simulink model "rtp_vector"  (R2024a)
settings: Solver=VariableStepAuto  StartTime=0.0  StopTime=4096*2  RelTol=1e-3
PostLoadFcn:
  | load filters
values from neighbouring files (symbols this model uses):
  narrow_filter = [180 89 -80 -391 -720 -834 -478 505 2063 3896 5535 6504]    [filters.mat]
  wide_filter = [-21 -249 319 -78 -511 977 -610 -844 2574 -2754 -1066 18539]    [filters.mat]
undefined symbols (not defined in the file or in its folder): None, S, vsva2197, xcvc1902
libraries: aieDSP x1, simulink x1, vmcUtilities x1, aieUtilities x1, dspobslib x1
settings Model: PauseTimes=511  Creator=abehbood  LastModifiedBy=robg
settings SolverCC: AlgebraicLoopSolver=TrustRegion
settings DebuggingCC: UnconnectedInputMsg=warning  UnconnectedOutputMsg=warning  UnconnectedLineMsg=warning
settings ModelReferenceCC: EnableRefExpFcnMdlSchedulingChecks=on
settings RTWCC: GPUComputeCapability=3.5  DLArmComputeVersion=19.05

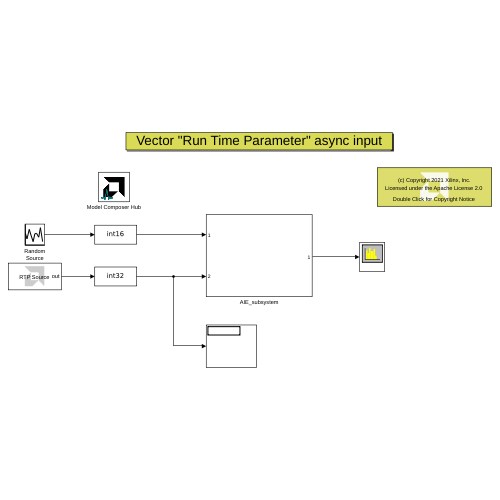
[thumbnail: Simulink's stored preview of the top-level diagram]
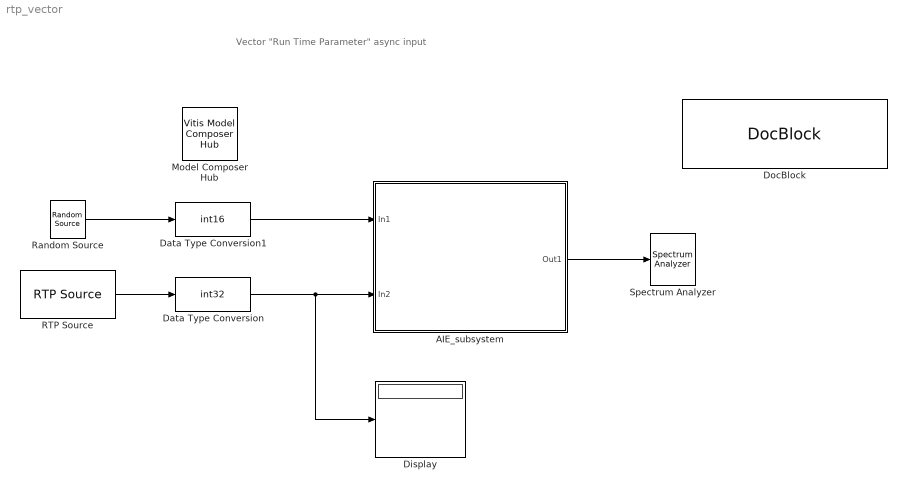
== system rtp_vector ==
  note: Vector "Run Time Parameter" async input
  AIE_subsystem : Subsystem
  Data Type Conversion : DataTypeConversion  OutDataTypeStr=int32  SaturateOnIntegerOverflow=off  RndMeth=Floor
  Data Type Conversion1 : DataTypeConversion  OutDataTypeStr=int16  SaturateOnIntegerOverflow=off  RndMeth=Floor
  Display : Display
  DocBlock : simulink/Model-Wide Utilities/DocBlock  DocumentType=Text  mask(DocBlock){}
      content=|
      | ///////////////////////////////////////////////////////////////////////////
      | // Copyright 2021 Xilinx
      | //
      | // Licensed under the Apache License, Version 2.0 (the "License");
      | // you may not use this file except in compliance with the License.
      | // You may obtain a copy of the License at
      | //
      | // http://www.apache.org/licenses/LICENSE-2.0
      | //
      | // Unless required by applicable law or agreed to in writing, software
      | // distributed under the License is distributed on an "AS IS" BASIS,
      | // WITHOUT WARRANTIES OR CONDITIONS OF ANY KIND, either express or implied.
      | // See the License for the specific language governing permissions and
      | // limitations under the License.
      | ///////////////////////////////////////////////////////////////////////////
      mask Display:
      | xmcDrawBlockIcon();
      | disp(['{\fontsize{10pt}(c) Copyright 2021' ' Xilinx, Inc.}\newline \newline '],'texmode','on');
      | disp('{\fontsize{10pt}Licensed under the Apache License 2.0}','texmode','on');
      | disp('\newline \newline \newline{\fontsize{10pt}Double Click for Copyright Notice}','texmode','on');
  Model Composer Hub : vmcUtilities/Vitis Model Composer Hub  Tag=genX  CodeGeneration=off  SubsystemName=AIE_subsystem  StartColumn=1  NumberOfColumns=1  TargetDirectory=./code  exportDesign=off  analyzeDesign=off  validateDesignOnHw=off  ExportType=AI Engines  IpVendor=xilinx.com  IpLibrary=hls  IpVersion=1.0  IpHWLanguage=Verilog  AieCompilerOptions={}  AieSimulatorOptions={}  CreateTestbench=on  TestbenchStackSize=10  RunRtlSim=off  RunCSim=off  RunAieSim=on  AieSimTimeout=50000  RunAieSimProfiling=off  LaunchVitisAnalyzer=off  PlotOutput=off  RunX86Sim=off  X86SimTimeout=10  GenHwImage=off  GenLibadfXo=off  GenHwValidationCode=off  PlatformType=Not Specified  HwSystemType=Baremetal  HwValidationTarget=hw  ProjDevice=xcvc1902-vsva2197-1LP-e-S  ProjDevicePart=xcvc1902-vsva2197-1LP-e-S  AIEType=AIE  SamplePeriod=-1  ClockFrequency=200  DataPathParallelism=1  xilinxfamily=versalaicore  part=xcvc1902  speed=-1LP-e-S  package=vsva2197  directory=./netlist  testbench=off  incr_netlist=off  synthesis_tool=Vivado  clock_wrapper=Clock Enables  dbl_ovrd=According to Block Masks  dcm_input_clock_period=10  sysclk_period=10  simulink_period=1  eval_field=0  LogFileName=/proj/xsjhdstaff4/abehbood/vmc_examples/gitent/Examples/AIENGINE/Run_Time_Parameters/rtp_vector/code/model_composer.log  NThreads=4
  RTP Source : aieUtilities/RTP Source  Value=[narrow_filter, nan(length(narrow_filter),500), wide_filter, nan(length(narrow_filter),500) ]  SampleTime=-1  OutputForm=Cyclic repetition
  Random Source : dspobslib/Random Source  SrcType=Uniform  NormMethod=Ziggurat  CltLength=12  MinVal=-1  MaxVal=1  MeanVal=0  VarVal=1  RepMode=Not repeatable  rawSeed=1  IsInherit=off  SampMode=Discrete  SampTime=1/64  SampFrame=64  DataType=Double  OutComplex=Complex  OutputFrames=off
  Spectrum Analyzer : SpectrumAnalyzer  WindowPosition=[1296 264 1006 450]  Visible=on  Method=Welch  SampleRate=64  Span=64  StartFrequency=-32  StopFrequency=32  AveragingMethod=Running  ForgettingFactor=0.5  YLimits=[-47.9713,75.3227]  AllowFFTLengthLessThanSamplesPerUpdate=on
  wires:
  Data Type Conversion/1 -> Display/1, AIE_subsystem/2(In2)
  RTP Source/1 -> Data Type Conversion/1
  Random Source/1 -> Data Type Conversion1/1
  Data Type Conversion1/1 -> AIE_subsystem/1(In1)
  AIE_subsystem/1(Out1) -> Spectrum Analyzer/1

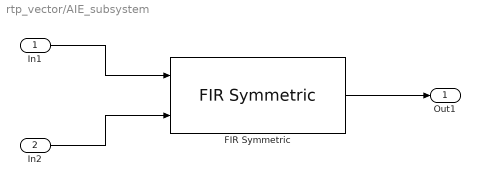
== system rtp_vector/AIE_subsystem ==
  In1 : Inport
  In2 : Inport  Port=2
  FIR Symmetric : aieDSP/FIR Symmetric  data_type=cint16  coef_type=int32  use_coeff_reload=on  dual_ip=off  num_outputs=off  coeff=[1, zeros(1,15)]  fir_length=24  input_window_size=64  shift_val=9  rnd_mode=Round to positive infinity  sat_mode=0-None  casc_length=1  AIE_VARIANT=1  TP_API=0  ssr=1  blockJsonConstraints=[]  blockJsonConstraintsInternal=[]  spec=vmc_fir_sr_sym.json  SerializedMaskParamNames=[]  SerializedMaskParamValues=[]  SerializedMaskParamVisibilities=[]  block_type=FIR Symmetric  SerializedMaskParamDataypes=typename|typename|uint|uint|uint|coef_type|uint|uint|uint|uint|uint|uint|uint|uint|uint  SerializedMaskParamEnumStrArr=0|0|0|0|0|0|0|0|0|Floor,Ceiling,Round to positive infinity,Round to negative infinity,Round symmetrical to infinity,Round symmetrical to zero,Round convergent to even,Round convergent to odd|0-None,1-Asymmetric,3-Symmetric|0|0|0|0  SerializedMaskParamEnumValArr=0|0|0|0|0|0|0|0|0|0,1,2,3,4,5,6,7|0,1,3|0|0|0|0  SerializedMaskParamVectorArr=0|0|0|0|0|1|0|0|0|0|0|0|0|0|0  SerializedMaskParamKeys=TT_DATA|TT_COEFF|TP_USE_COEFF_RELOAD|TP_DUAL_IP|TP_NUM_OUTPUTS|coeff|TP_FIR_LEN|TP_INPUT_WINDOW_VSIZE|TP_SHIFT|TP_RND|TP_SAT|TP_CASC_LEN|AIE_VARIANT|TP_API|TP_SSR
  Out1 : Outport
  wires:
  In2/1 -> FIR Symmetric/2
  In1/1 -> FIR Symmetric/1
  FIR Symmetric/1 -> Out1/1
